simulink model "simu_intern_model"  (R2023a)
settings: Solver=VariableStepAuto  StartTime=0.0  StopTime=0.1  RelTol=1e-3
undefined symbols (not defined in the file): Az_I, Bz_I, Cz_I, Fz_I, Gz_I, Te
settings Model: Creator=sfahim  LastModifiedBy=sfahim

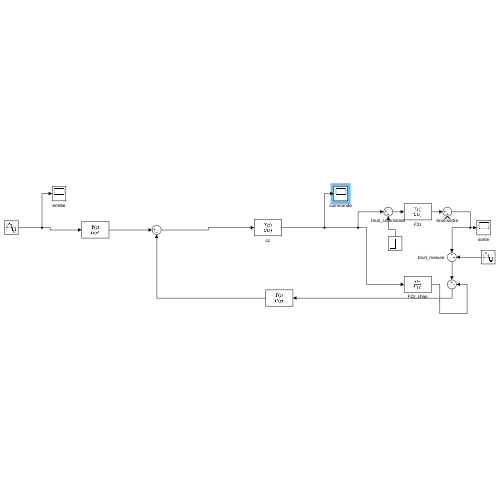
[thumbnail: Simulink's stored preview of the top-level diagram]
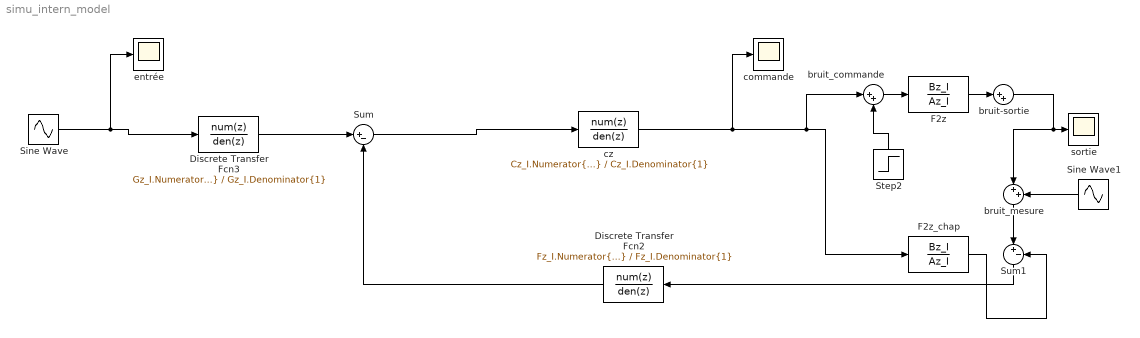
== system simu_intern_model ==
  Discrete Transfer Fcn2 : DiscreteTransferFcn  Numerator=Fz_I.Numerator{1}  Denominator=Fz_I.Denominator{1}  SampleTime=Te
  Discrete Transfer Fcn3 : DiscreteTransferFcn  Numerator=Gz_I.Numerator{1}  Denominator=Gz_I.Denominator{1}  SampleTime=Te
  F2z : DiscreteTransferFcn  Numerator=Bz_I  Denominator=Az_I  SampleTime=Te
  F2z_chap : DiscreteTransferFcn  Numerator=Bz_I  Denominator=Az_I  SampleTime=Te
  Sine Wave : Sin  Amplitude=25  Frequency=314  SampleTime=Te
  Sine Wave1 : Sin  Frequency=9500  SampleTime=Te
  Step2 : Step  Time=0.05  SampleTime=Te
  Sum : Sum  Inputs=|+-
  Sum1 : Sum  Inputs=|+-
  bruit-sortie : Sum  Inputs=|++
  bruit_commande : Sum  Inputs=|++
  bruit_mesure : Sum  Inputs=|++
  commande : Scope
  cz : DiscreteTransferFcn  Numerator=Cz_I.Numerator{1}  Denominator=Cz_I.Denominator{1}  SampleTime=Te
  entrée : Scope
  sortie : Scope
  wires:
  cz/1 -> commande/1, bruit_commande/1, F2z_chap/1
  Sum/1 -> cz/1
  Discrete Transfer Fcn2/1 -> Sum/2
  F2z_chap/1 -> Sum1/2
  Sum1/1 -> Discrete Transfer Fcn2/1
  Discrete Transfer Fcn3/1 -> Sum/1
  Sine Wave/1 -> entrée/1, Discrete Transfer Fcn3/1
  bruit_mesure/1 -> Sum1/1
  bruit_commande/1 -> F2z/1
  F2z/1 -> bruit-sortie/1
  bruit-sortie/1 -> bruit_mesure/1, sortie/1
  Sine Wave1/1 -> bruit_mesure/2
  Step2/1 -> bruit_commande/2
